simulink model "real_double_pendulum"  (R2024a)
settings: Solver=VariableStepAuto  StartTime=0.0  StopTime=30  RelTol=1e-3
libraries: fl_lib x44, ee_lib x19, nesl_utility x3
settings DataIOCC: ReturnWorkspaceOutputs=off

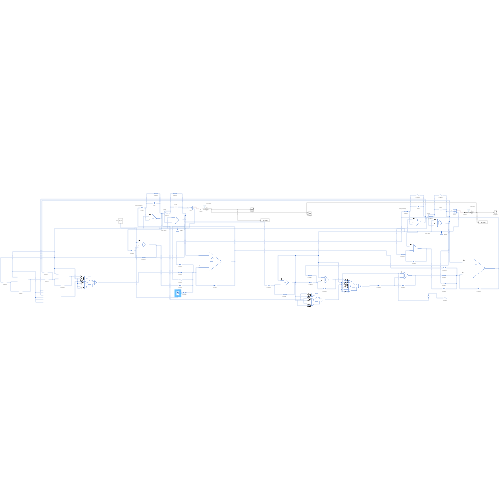
[thumbnail: Simulink's stored preview of the top-level diagram]
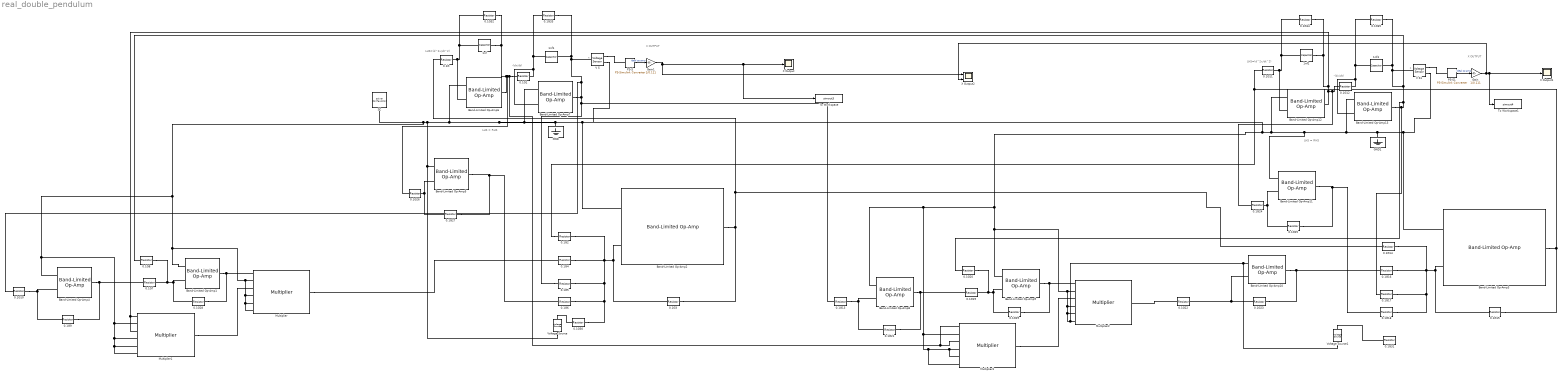
== system real_double_pendulum ==
  note: X OUTPUT
  note: LHS=(d^2x/dt^2)
  note: -(dx/dt)
  note: LHS = RHS
  note: -(dx/dt)
  note: LHS = RHS
  note: x
  note: X OUTPUT
  note: x
  note: LHS=(d^2x/dt^2)
  0.1G{,1,11..12,32..35} (8 alike) : fl_lib/Electrical/Electrical Elements/Resistor  R=1 GOhm  i_specify=off  i_priority=None  i=0 A  i_nominal_specify=off  i_nominal_value=1  i_nominal_unit=A  v_specify=off  v_priority=None  v=0 V  v_nominal_specify=off  v_nominal_value=1  v_nominal_unit=V
  0.1G{3,7..10,13,15,19..31} (20 alike) : fl_lib/Electrical/Electrical Elements/Resistor  R=10 kOhm  i_specify=off  i_priority=None  i=0 A  i_nominal_specify=off  i_nominal_value=1  i_nominal_unit=A  v_specify=off  v_priority=None  v=0 V  v_nominal_specify=off  v_nominal_value=1  v_nominal_unit=V
  0.1G14 : fl_lib/Electrical/Electrical Elements/Resistor  R=6.67 kOhm  i_specify=off  i_priority=None  i=0 A  i_nominal_specify=off  i_nominal_value=1  i_nominal_unit=A  v_specify=off  v_priority=None  v=0 V  v_nominal_specify=off  v_nominal_value=1  v_nominal_unit=V
  0.1G16 : fl_lib/Electrical/Electrical Elements/Resistor  R=6.67 kOhm  i_specify=off  i_priority=None  i=0 A  i_nominal_specify=off  i_nominal_value=1  i_nominal_unit=A  v_specify=off  v_priority=None  v=0 V  v_nominal_specify=off  v_nominal_value=1  v_nominal_unit=V
  0.1G17 : fl_lib/Electrical/Electrical Elements/Resistor  R=0.67958 kOhm  i_specify=off  i_priority=None  i=0 A  i_nominal_specify=off  i_nominal_value=1  i_nominal_unit=A  v_specify=off  v_priority=None  v=0 V  v_nominal_specify=off  v_nominal_value=1  v_nominal_unit=V
  0.1G18 : fl_lib/Electrical/Electrical Elements/Resistor  R=3.33 kOhm  i_specify=off  i_priority=None  i=0 A  i_nominal_specify=off  i_nominal_value=1  i_nominal_unit=A  v_specify=off  v_priority=None  v=0 V  v_nominal_specify=off  v_nominal_value=1  v_nominal_unit=V
  0.1G2 : fl_lib/Electrical/Electrical Elements/Resistor  R=33.33 kOhm  i_specify=off  i_priority=None  i=0 A  i_nominal_specify=off  i_nominal_value=1  i_nominal_unit=A  v_specify=off  v_priority=None  v=0 V  v_nominal_specify=off  v_nominal_value=1  v_nominal_unit=V
  0.1G4 : fl_lib/Electrical/Electrical Elements/Resistor  R=33.33 kOhm  i_specify=off  i_priority=None  i=0 A  i_nominal_specify=off  i_nominal_value=1  i_nominal_unit=A  v_specify=off  v_priority=None  v=0 V  v_nominal_specify=off  v_nominal_value=1  v_nominal_unit=V
  0.1G5 : fl_lib/Electrical/Electrical Elements/Resistor  R=0.84947 kOhm  i_specify=off  i_priority=None  i=0 A  i_nominal_specify=off  i_nominal_value=1  i_nominal_unit=A  v_specify=off  v_priority=None  v=0 V  v_nominal_specify=off  v_nominal_value=1  v_nominal_unit=V
  0.1G6 : fl_lib/Electrical/Electrical Elements/Resistor  R=16.67 kOhm  i_specify=off  i_priority=None  i=0 A  i_nominal_specify=off  i_nominal_value=1  i_nominal_unit=A  v_specify=off  v_priority=None  v=0 V  v_nominal_specify=off  v_nominal_value=1  v_nominal_unit=V
  1nf : fl_lib/Electrical/Electrical Elements/Capacitor  c=1e-09 F  r=1e-06 Ohm  g=0 1/Ohm  i_specify=off  i_priority=None  i=0 A  i_nominal_specify=off  i_nominal_value=1  i_nominal_unit=A  v_specify=off  v_priority=None  v=4 V  v_nominal_specify=off  v_nominal_value=1  v_nominal_unit=V  vc_specify=off  vc_priority=High  vc=0 V  vc_nominal_specify=off  vc_nominal_value=1  vc_nominal_unit=V
  1nf1 : fl_lib/Electrical/Electrical Elements/Capacitor  c=1e-09 F  r=1e-06 Ohm  g=0 1/Ohm  i_specify=off  i_priority=None  i=0 A  i_nominal_specify=off  i_nominal_value=1  i_nominal_unit=A  v_specify=off  v_priority=None  v=20 V  v_nominal_specify=off  v_nominal_value=1  v_nominal_unit=V  vc_specify=off  vc_priority=High  vc=-2.22 V  vc_nominal_specify=off  vc_nominal_value=1  vc_nominal_unit=V
  1nf2 : fl_lib/Electrical/Electrical Elements/Capacitor  c=1e-09 F  r=1e-06 Ohm  g=0 1/Ohm  i_specify=off  i_priority=None  i=0 A  i_nominal_specify=off  i_nominal_value=1  i_nominal_unit=A  v_specify=off  v_priority=None  v=4 V  v_nominal_specify=off  v_nominal_value=1  v_nominal_unit=V  vc_specify=off  vc_priority=High  vc=0 V  vc_nominal_specify=off  vc_nominal_value=1  vc_nominal_unit=V
  1nf3 : fl_lib/Electrical/Electrical Elements/Capacitor  c=1e-09 F  r=1e-06 Ohm  g=0 1/Ohm  i_specify=off  i_priority=None  i=0 A  i_nominal_specify=off  i_nominal_value=1  i_nominal_unit=A  v_specify=off  v_priority=None  v=20 V  v_nominal_specify=off  v_nominal_value=1  v_nominal_unit=V  vc_specify=off  vc_priority=High  vc=-2.23221 V  vc_nominal_specify=off  vc_nominal_value=1  vc_nominal_unit=V
  Band-Limited Op-Amp{1..13} (13 alike) : ee_lib/Integrated Circuits/Band-Limited Op-Amp  A=1.8e6  Rin=20 MOhm  Rout=70 Ohm  Vmin=-12 V  Vmax=12 V  Vdotmax=20000000 V/s  f=20 MHz  V0=0 V
  GND : fl_lib/Electrical/Electrical Elements/Electrical Reference
  GND1 : fl_lib/Electrical/Electrical Elements/Electrical Reference
  Gain : Gain  Gain=1/0.111
  Gain1 : Gain  Gain=1/0.111
  Multiplier{,1..3} (4 alike) : ee_lib/Integrated Circuits/Multiplier  K=1 V  A=1  Rin=10e6 Ohm  Vdiff=10 V  Rout=0.1 Ohm  Vmin=-11 V  Vmax=11 V  Vdotmax=20 V/us  f=1 MHz  V0=0 V
      settings: InternalSimscapePortConfiguration="{\"Bottom\":[],\"Left\":[{\"id\":\"X1\",\"label\":\"X1\",\"type\":\"foundation.electrical.electrical\"},{\"id\":\"X2\",\"label\":\"X2\",\"type\":\"foundation.electrical.electrical\"},{\"id\":\"Y1\",\"label\":\"Y1\",\"type\":\"foundation.electrical.electrical\"},{\"id\":\"Y2\",\"label\":\"Y2\",\"type\":\"foundation.electrical.electrical\"},{\"id\":\"Z1\",\"label\":\"Z1\",\"type\":\"foundation.electrical.electrical\"},{\"id\":\"Z2\",\"label\":\"Z2\",\"type\":\"foundation.electrical.electrical\"}],\"Right\":[{\"id\":\"out\",\"label\":\"\",\"type\":\"foundation.electrical.electrical\"}],\"Top\":[]}"
  PS-S : nesl_utility/PS-Simulink Converter  PhysicalDomain=network_engine_domain  SubClassName=ps_output  LeftPortType=input  RightPortType=output  PseudoPeriodic=off  Frequencies=[]  VectorFormat=1-D array  Unit=1  AffineConversion=off
  PS-S1 : nesl_utility/PS-Simulink Converter  PhysicalDomain=network_engine_domain  SubClassName=ps_output  LeftPortType=input  RightPortType=output  PseudoPeriodic=off  Frequencies=[]  VectorFormat=1-D array  Unit=1  AffineConversion=off
  SC : nesl_utility/Solver Configuration  PhysicalDomain=network_engine_domain  SubClassName=solver  LeftPortType=input  RightPortType=generic  Tones=[]  Harmonics=[]  SimulateNoise=off  Profile=off  UseLocalSampling=off  EnableSwitchedLinearOptims=on  FrequencyDomain=off  UseCCode=off  RelTol=0.001  AbsTol=0.001  MinStep=1e-09  ToWorkspace=off  RevertToSquareIcSolve=off  NumHomotopyIterations=100  PhasorMode=off  PhasorModeNumHarmonics=1  ConsistencySolver=NEWTON_FTOL  IndexReductionMethod=DerivativeReplacement  DoDC=off  ResidualTolerance=1e-9  ConsistencyTolSource=GLOBAL  ConsistencyAbsTol=0.001  ConsistencyRelTol=0.001  ConsistencyTolFactor=0.001  UseLocalSolver=off  LocalSolverChoice=NE_BACKWARD_EULER_ADVANCER  ResolveIndetEquations=on  FunctionEvalNumThread=1  LocalSolverSampleTime=0.001  DoFixedCost=off  MaxNonlinIter=12  MaxModeIter=2  ComputeImpulses=off  ImpulseIterations=2  LinearAlgebra=Sparse  LinearAlgebraNumThread=0  EquationFormulation=NE_TIME_EF  DelaysMemoryBudget=1024  AutomaticFiltering=on  FilteringTimeConstant=0.001  PartitionStorageMethod=AS_NEEDED  PartitionMemoryBudget=1024  PartitionMethod=FAST  MultibodyUseLocalSolver=on  MultibodyLocalSolverChoice=ODE1  MultibodyLocalSolverSampleTime=0.001
  To Workspace : ToWorkspace  VariableName=simout3  SampleTime=0.001
      settings: Save2DSignal=2-D array (concatenate along first dimension)
  To Workspace1 : ToWorkspace  VariableName=simout4  SampleTime=0.001
      settings: Save2DSignal=2-D array (concatenate along first dimension)
  V S : fl_lib/Electrical/Electrical Sensors/Voltage Sensor
  V S1 : fl_lib/Electrical/Electrical Sensors/Voltage Sensor
  Voltage Source : ee_lib/Sources/Voltage Source  dc_voltage=11 V  ac_voltage=0 V  ac_shift=0 rad  ac_frequency=60 Hz  noise_mode=ee.enum.sources.noise.Disabled  PSD=0 V^2/Hz  sample_time=1e-3 s  repeatability=ee.enum.sources.repeatability.NotRepeatable  user_seed=0  auto_seed=3499211588  i_specify=off  i_priority=None  i=0 A  i_nominal_specify=off  i_nominal_value=1  i_nominal_unit=A  v_specify=off  v_priority=None  v=0 V  v_nominal_specify=off  v_nominal_value=1  v_nominal_unit=V
  Voltage Source1 : ee_lib/Sources/Voltage Source  dc_voltage=1 V  ac_voltage=0 V  ac_shift=0 rad  ac_frequency=60 Hz  noise_mode=ee.enum.sources.noise.Disabled  PSD=0 V^2/Hz  sample_time=1e-3 s  repeatability=ee.enum.sources.repeatability.NotRepeatable  user_seed=0  auto_seed=3890346746  i_specify=off  i_priority=None  i=0 A  i_nominal_specify=off  i_nominal_value=1  i_nominal_unit=A  v_specify=off  v_priority=None  v=0 V  v_nominal_specify=off  v_nominal_value=1  v_nominal_unit=V
  X Output : Scope
  X Output1 : Scope
  X Output2 : Scope  NumInputPorts=2
  wires:
  PS-S/1 -> Gain1/1  "Ideal op amp"
  PS-S1/1 -> Gain/1  "Ideal op amp"
  Gain1/1 -> To Workspace/1, X Output/1, X Output2/1
  Gain/1 -> X Output1/1, To Workspace1/1, X Output2/2
  connections:
  V S/RConn2 -- Band-Limited Op-Amp2/LConn1 -- Band-Limited Op-Amp7/LConn1 -- Band-Limited Op-Amp8/LConn1 -- Multiplier3/LConn6 -- Multiplier3/LConn5 -- Multiplier3/LConn4 -- Multiplier3/LConn2 -- Band-Limited Op-Amp9/LConn1 -- Voltage Source1/RConn1 -- Band-Limited Op-Amp10/LConn1 -- Multiplier2/LConn6 -- Multiplier2/LConn5 -- Multiplier2/LConn4 -- Multiplier2/LConn2 -- Band-Limited Op-Amp12/LConn1 -- Band-Limited Op-Amp11/LConn1 -- Band-Limited Op-Amp13/LConn1 -- GND1/LConn1 -- Band-Limited Op-Amp3/LConn1 -- V S1/RConn2 -- Band-Limited Op-Amp6/LConn1 -- Voltage Source/RConn1 -- Band-Limited Op-Amp5/LConn1 -- Band-Limited Op-Amp1/LConn1 -- Multiplier/LConn6 -- Multiplier/LConn5 -- Multiplier/LConn4 -- Multiplier/LConn2 -- Band-Limited Op-Amp4/LConn1 -- Multiplier1/LConn6 -- Multiplier1/LConn5 -- Multiplier1/LConn4 -- Multiplier1/LConn2 -- SC/RConn1 -- GND/LConn1
  0.1G29/LConn1 -- Band-Limited Op-Amp9/LConn2 -- 0.1G20/RConn1 -- 0.1G19/RConn1
  0.1G19/LConn1 -- Band-Limited Op-Amp8/RConn1 -- 0.1G21/RConn1
  0.1G15/LConn1 -- Band-Limited Op-Amp3/LConn2 -- 0.1G14/RConn1 -- 0.1G16/RConn1 -- 0.1G18/RConn1 -- 0.1G17/RConn1
  0.1G3/RConn1 -- Band-Limited Op-Amp2/RConn1 -- 0.1G/LConn1 -- 0.1G14/LConn1
  0.1G2/LConn1 -- Band-Limited Op-Amp3/RConn1 -- 0.1G15/RConn1 -- 0.1G11/LConn1
  0.1G22/RConn1 -- Band-Limited Op-Amp10/LConn2 -- 0.1G23/LConn1
  0.1G27/RConn1 -- Band-Limited Op-Amp5/RConn1 -- 0.1G6/LConn1
  0.1G27/LConn1 -- Band-Limited Op-Amp5/LConn2 -- 0.1G26/RConn1
  0.1G23/RConn1 -- Band-Limited Op-Amp10/RConn1 -- 0.1G16/LConn1
  0.1G1/LConn1 -- Multiplier3/LConn3 -- Multiplier3/LConn1 -- 0.1G26/LConn1 -- 0.1G32/RConn1 -- 1nf/RConn1 -- Band-Limited Op-Amp6/RConn1
  0.1G9/LConn1 -- Band-Limited Op-Amp4/LConn2 -- 0.1G10/RConn1
  0.1G13/RConn1 -- Band-Limited Op-Amp8/LConn2 -- 0.1G21/LConn1
  0.1G5/LConn1 -- Band-Limited Op-Amp7/RConn1 -- 0.1G10/LConn1 -- 0.1G33/RConn1 -- 1nf1/RConn1 -- V S/LConn1 -- 0.1G13/LConn1
  1nf3/RConn1 -- 0.1G8/LConn1 -- 0.1G20/LConn1 -- Band-Limited Op-Amp13/RConn1 -- 0.1G17/LConn1 -- V S1/LConn1 -- 0.1G35/RConn1
  0.1G28/RConn1 -- Band-Limited Op-Amp1/RConn1 -- Multiplier/LConn1
  0.1G1/RConn1 -- Band-Limited Op-Amp7/LConn2 -- 0.1G33/LConn1 -- 1nf1/LConn1
  0.1G25/RConn1 -- Band-Limited Op-Amp11/RConn1 -- 0.1G18/LConn1
  Band-Limited Op-Amp13/LConn2 -- 0.1G12/RConn1 -- 0.1G35/LConn1 -- 1nf3/LConn1
  0.1G29/RConn1 -- Band-Limited Op-Amp9/RConn1 -- Multiplier2/LConn1
  0.1G/RConn1 -- Band-Limited Op-Amp6/LConn2 -- 0.1G32/LConn1 -- 1nf/LConn1
  0.1G9/RConn1 -- Band-Limited Op-Amp4/RConn1 -- 0.1G7/LConn1
  0.1G4/RConn1 -- Band-Limited Op-Amp2/LConn2 -- 0.1G3/LConn1 -- 0.1G2/RConn1 -- 0.1G30/RConn1 -- 0.1G6/RConn1 -- 0.1G5/RConn1
  Multiplier1/LConn1 -- 0.1G34/RConn1 -- 1nf2/RConn1 -- Band-Limited Op-Amp12/RConn1 -- 0.1G24/LConn1 -- 0.1G12/LConn1 -- Multiplier1/LConn3
  0.1G7/RConn1 -- Band-Limited Op-Amp1/LConn2 -- 0.1G28/LConn1 -- 0.1G8/RConn1
  0.1G24/RConn1 -- Band-Limited Op-Amp11/LConn2 -- 0.1G25/LConn1
  Band-Limited Op-Amp12/LConn2 -- 0.1G11/RConn1 -- 0.1G34/LConn1 -- 1nf2/LConn1
  V S1/RConn1 -- PS-S1/LConn1
  Multiplier3/RConn1 -- Multiplier2/LConn3
  Multiplier1/RConn1 -- Multiplier/LConn3
  0.1G22/LConn1 -- Multiplier2/RConn1
  V S/RConn1 -- PS-S/LConn1
  Multiplier/RConn1 -- 0.1G4/LConn1
  0.1G30/LConn1 -- Voltage Source/LConn1
  0.1G31/LConn1 -- Voltage Source1/LConn1
